simulink model "sampleModel1570_3"  (R2023a)
settings: Solver=VariableStepAuto  StartTime=0.0  StopTime=10.0  RelTol=1e-3
libraries: hdlsllib x8, simulink x3
settings Model: Creator=user1  LastModifiedBy=user1

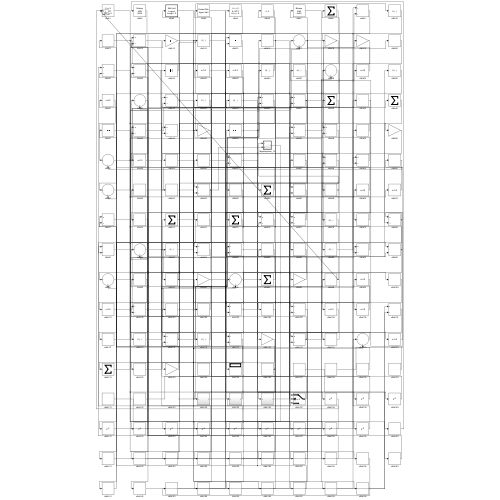
[thumbnail: Simulink's stored preview of the top-level diagram]
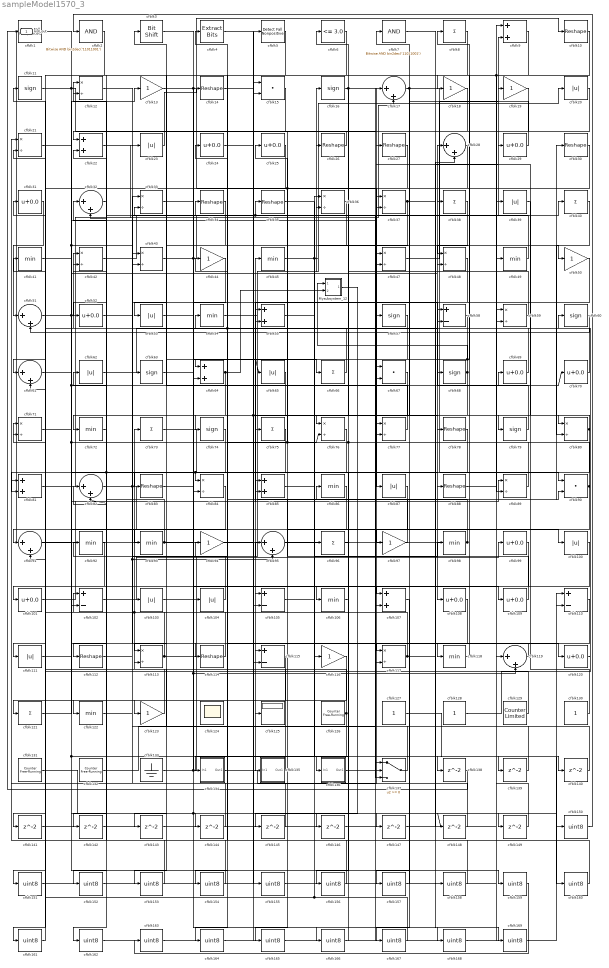
== system sampleModel1570_3 ==
  Mysubsystem_12 : Subsystem  TreatAsAtomicUnit=on  RTWFcnName=Mysubsystem_12
      settings: RTWFcnNameOpts=User specified  RTWFileNameOpts=Use function name
  cfblk1 : hdlsllib/Logic and Bit Operations/Detect Fall Nonpositive  vinit=0  OutDataTypeStr=uint8
  cfblk{10,14,26..27,30,34..35,78,83,88,112,114} (12 alike) : Reshape
  cfblk{20,23,39,53,62,65,87,100,103..104,111} (11 alike) : Abs  OutDataTypeStr=uint8  SaturateOnIntegerOverflow=off
  cfblk{24..25,29,31,52,69..70,99,101,108..109,120} (12 alike) : Bias  Bias=0.0  SaturateOnIntegerOverflow=off
  cfblk{58,102,105,110,115} (5 alike) : Sum  Inputs=+-  OutDataTypeStr=uint8
  cfblk{41,45,49,54,72,86,92..93,98,106,118,122} (12 alike) : MinMax  OutDataTypeStr=uint8
  cfblk{9,22,55,64,81,85,107} (7 alike) : Sum  OutDataTypeStr=uint8
  cfblk{11,16,57,60,63,68,74,79} (8 alike) : Signum
  cfblk{12,21,33,36..37,42..43,47..48,59,71,76..77,80,84,89,113,117} (18 alike) : Product  Inputs=*/  OutDataTypeStr=uint8  RndMeth=Zero  SaturateOnIntegerOverflow=on
  cfblk{13,18..19,44,50,94,97,116,123} (9 alike) : Gain  OutDataTypeStr=uint8
  cfblk{17,28,32,51,61,82,91,95,119} (9 alike) : Sum  Inputs=|++  OutDataTypeStr=uint8
  cfblk{8,38,40,66,73,75,96,121} (8 alike) : Sum  Inputs=+  OutDataTypeStr=uint8
  cfblk124 : Scope
      settings: Floating=on
  cfblk125 : Display
  cfblk126 : hdlsllib/Sources/Counter Free-Running  NumBits=16  tsamp=-1
  cfblk127 : Constant  OutDataTypeStr=uint8  SampleTime=-1
  cfblk128 : Constant  OutDataTypeStr=uint8  SampleTime=-1
  cfblk129 : hdlsllib/Sources/Counter Limited  uplimit=7  tsamp=-1
  cfblk130 : Constant  OutDataTypeStr=uint8  SampleTime=-1
  cfblk131 : hdlsllib/Sources/Counter Free-Running  NumBits=16  tsamp=-1
  cfblk132 : hdlsllib/Sources/Counter Free-Running  NumBits=16  tsamp=-1
  cfblk133 : Ground
  cfblk134 : Subsystem
      settings: LibrarySourceBlock=|
      | hdlsllib/Ports &
      | Subsystems/Subsystem
  cfblk135 : Subsystem
      settings: LibrarySourceBlock=|
      | hdlsllib/Ports &
      | Subsystems/Subsystem
  cfblk136 : Subsystem
      settings: LibrarySourceBlock=|
      | hdlsllib/Ports &
      | Subsystems/Subsystem
  cfblk137 : Switch  OutDataTypeStr=uint8  SaturateOnIntegerOverflow=off  InputSameDT=off
  cfblk{138..149} (12 alike) : Delay  SampleTime=1
  cfblk15 : DotProduct  OutDataTypeStr=uint8
  cfblk{150..169} (20 alike) : DataTypeConversion  OutDataTypeStr=uint8  SaturateOnIntegerOverflow=off  RndMeth=Floor
  cfblk2 : simulink/Logic and Bit Operations/Bitwise Operator  logicop=AND  UseBitMask=on  BitMask=bin2dec('11011001')  BitMaskRealWorld=Stored Integer
      settings: LibrarySourceBlock=|
      | hdlsllib/Logic and Bit
      | Operations/Bitwise
      | Operator
  cfblk3 : hdlsllib/Logic and Bit Operations/Bit Shift  mode=Shift Left Logical  N=0
  cfblk4 : simulink/Logic and Bit Operations/Extract Bits  bitsToExtract=Upper half  numBits=8  bitIdxRange=[0 7]  outScalingMode=Preserve fixed-point scaling
      settings: LibrarySourceBlock=|
      | hdlsllib/Logic and Bit
      | Operations/Extract Bits
  cfblk5 : hdlsllib/Logic and Bit Operations/Detect Fall Nonpositive  vinit=0  OutDataTypeStr=uint8
  cfblk6 : hdlsllib/Logic and Bit Operations/Compare To Constant  relop=<=  const=3.0  OutDataTypeStr=uint8
  cfblk67 : DotProduct  OutDataTypeStr=uint8
  cfblk7 : simulink/Logic and Bit Operations/Bitwise Operator  logicop=AND  UseBitMask=on  BitMask=bin2dec('11011001')  BitMaskRealWorld=Stored Integer
      settings: LibrarySourceBlock=|
      | hdlsllib/Logic and Bit
      | Operations/Bitwise
      | Operator
  cfblk90 : DotProduct  OutDataTypeStr=uint8
  Hdl_out : Outport  OutDataTypeStr=uint8
  wires:
  cfblk135/1(Out1) -> cfblk73/1
  cfblk134/1(Out1) -> cfblk17/1
  cfblk98/1 -> cfblk45/1, Hdl_out/1
  cfblk34/1 -> cfblk93/1
  cfblk29/1 -> cfblk64/1
  cfblk97/1 -> cfblk34/1
  cfblk75/1 -> cfblk82/2, cfblk91/1, cfblk84/1
  cfblk19/1 -> cfblk113/1
  cfblk17/1 -> cfblk90/1, cfblk77/1
  cfblk133/1 -> cfblk16/1, cfblk58/2
  cfblk101/1 -> cfblk89/1
  cfblk23/1 -> cfblk10/1
  cfblk13/1 -> cfblk87/1, cfblk137/2
  cfblk93/1 -> cfblk109/1, cfblk12/2
  cfblk45/1 -> cfblk50/1, cfblk78/1
  cfblk90/1 -> cfblk25/1, cfblk6/1, cfblk146/1
  cfblk48/1 -> cfblk135/1(In1)
  cfblk73/1 -> cfblk125/1
  cfblk128/1 -> cfblk80/1
  cfblk3/1 -> cfblk148/1, cfblk168/1, cfblk119/2
  cfblk49/1 -> cfblk35/1, cfblk12/1
  cfblk54/1 -> cfblk20/1
  cfblk99/1 -> cfblk101/1
  cfblk8/1 -> cfblk18/1
  cfblk43/1 -> cfblk9/2, cfblk37/1
  cfblk25/1 -> cfblk53/1
  cfblk89/1 -> cfblk4/1, cfblk55/2
  cfblk47/1 -> cfblk19/1
  cfblk83/1 -> cfblk14/1
  cfblk88/1 -> cfblk49/1
  cfblk113/1 -> cfblk103/1, cfblk91/2, cfblk26/1
  cfblk81/1 -> cfblk23/1
  cfblk39/1 -> cfblk79/1
  cfblk102/1 -> cfblk99/1
  cfblk79/1 -> cfblk28/1
  cfblk80/1 -> cfblk72/1, cfblk136/1(In1)
  cfblk26/1 -> cfblk22/1
  cfblk42/1 -> cfblk5/1
  cfblk110/1 -> cfblk167/1
  cfblk116/1 -> cfblk121/1
  cfblk52/1 -> cfblk118/1
  cfblk114/1 -> cfblk102/1
  cfblk20/1 -> cfblk89/2
  cfblk5/1 -> cfblk61/1
  cfblk115/1 -> cfblk122/1
  cfblk100/1 -> cfblk106/1
  cfblk95/1 -> cfblk69/1
  cfblk64/1 -> Mysubsystem_12/2(In2), cfblk112/1
  cfblk50/1 -> cfblk108/1
  cfblk78/1 -> cfblk111/1
  cfblk30/1 -> cfblk115/1, cfblk61/2
  cfblk31/1 -> cfblk51/1
  cfblk111/1 -> cfblk70/1, cfblk37/2
  cfblk10/1 -> cfblk68/1
  cfblk51/1 -> cfblk17/2, cfblk88/1, cfblk13/1
  cfblk33/1 -> cfblk66/1
  cfblk109/1 -> cfblk85/1
  cfblk82/1 -> cfblk115/2, cfblk120/1
  cfblk69/1 -> cfblk42/1
  cfblk62/1 -> cfblk57/1
  cfblk77/1 -> cfblk3/1
  cfblk24/1 -> cfblk107/1, cfblk77/2
  cfblk59/1 -> cfblk33/2
  cfblk37/1 -> cfblk84/2, cfblk29/1
  cfblk57/1 -> cfblk74/1
  cfblk119/1 -> cfblk117/1
  cfblk28/1 -> cfblk67/1
  cfblk35/1 -> cfblk116/1
  cfblk103/1 -> cfblk30/1
  cfblk44/1 -> cfblk64/2
  cfblk105/1 -> cfblk98/1
  cfblk132/1 -> cfblk47/1
  cfblk71/1 -> cfblk97/1, cfblk76/2
  cfblk76/1 -> cfblk81/2
  cfblk96/1 -> cfblk36/2
  cfblk65/1 -> cfblk83/1
  cfblk123/1 -> cfblk71/1
  cfblk68/1 -> Mysubsystem_12/1(In1), cfblk65/1, cfblk75/1
  cfblk12/1 -> cfblk63/1
  cfblk16/1 -> cfblk137/1, cfblk76/1
  cfblk60/1 -> cfblk51/2
  cfblk11/1 -> cfblk137/3, cfblk147/1, cfblk117/2
  cfblk40/1 -> cfblk80/2
  cfblk58/1 -> cfblk123/1
  cfblk129/1 -> cfblk71/2
  cfblk38/1 -> cfblk48/1
  cfblk18/1 -> cfblk55/1
  cfblk130/1 -> cfblk27/1
  cfblk104/1 -> cfblk92/1
  cfblk136/1(Out1) -> cfblk38/1
  cfblk70/1 -> cfblk41/1, cfblk44/1
  cfblk121/1 -> cfblk85/2
  cfblk63/1 -> cfblk104/1
  cfblk112/1 -> cfblk95/1
  cfblk117/1 -> cfblk42/2, cfblk90/2
  cfblk120/1 -> cfblk60/1
  cfblk1/1 -> cfblk43/2, cfblk114/1
  cfblk9/1 -> cfblk52/1, cfblk59/2
  cfblk126/1 -> cfblk134/1(In1), cfblk31/1
  cfblk87/1 -> cfblk105/1
  cfblk66/1 -> cfblk24/1
  cfblk61/1 -> cfblk48/2
  cfblk122/1 -> cfblk95/2, cfblk40/1
  cfblk118/1 -> cfblk8/1
  cfblk92/1 -> cfblk102/2
  cfblk137/1 -> cfblk54/1
  cfblk22/1 -> cfblk58/1
  cfblk91/1 -> cfblk100/1
  cfblk67/1 -> cfblk105/2
  cfblk55/1 -> cfblk138/1
  cfblk138/1 -> cfblk1/1
  cfblk85/1 -> cfblk139/1
  cfblk139/1 -> cfblk33/1
  cfblk4/1 -> cfblk140/1
  cfblk140/1 -> cfblk113/2
  cfblk84/1 -> cfblk141/1
  cfblk141/1 -> cfblk9/1
  cfblk72/1 -> cfblk142/1
  cfblk142/1 -> cfblk22/2
  cfblk36/1 -> cfblk143/1
  cfblk143/1 -> cfblk28/2
  cfblk41/1 -> cfblk144/1
  cfblk144/1 -> cfblk43/1
  cfblk145/1 -> cfblk81/1
  cfblk146/1 -> cfblk107/2
  cfblk148/1 -> cfblk82/1
  cfblk14/1 -> cfblk149/1
  cfblk149/1 -> cfblk59/1
  cfblk127/1 -> cfblk150/1
  cfblk150/1 -> cfblk2/1
  cfblk2/1 -> cfblk151/1
  cfblk151/1 -> cfblk119/1
  cfblk32/1 -> cfblk152/1
  cfblk152/1 -> cfblk96/1
  cfblk6/1 -> cfblk153/1
  cfblk153/1 -> cfblk32/1
  cfblk108/1 -> cfblk154/1
  cfblk154/1 -> cfblk32/2
  cfblk94/1 -> cfblk155/1
  cfblk155/1 -> cfblk67/2
  cfblk106/1 -> cfblk156/1
  cfblk156/1 -> cfblk94/1
  cfblk107/1 -> cfblk157/1
  cfblk157/1 -> cfblk7/1
  cfblk7/1 -> cfblk158/1
  cfblk158/1 -> cfblk62/1
  cfblk21/1 -> cfblk159/1
  cfblk131/1 -> cfblk160/1
  cfblk160/1 -> cfblk21/1
  cfblk74/1 -> cfblk161/1
  cfblk161/1 -> cfblk21/2
  cfblk15/1 -> cfblk162/1
  cfblk162/1 -> cfblk47/2
  cfblk159/1 -> cfblk163/1
  cfblk163/1 -> cfblk15/1
  cfblk27/1 -> cfblk164/1
  cfblk164/1 -> cfblk15/2
  cfblk86/1 -> cfblk165/1
  cfblk165/1 -> cfblk39/1
  cfblk53/1 -> cfblk166/1
  cfblk166/1 -> cfblk86/1
  cfblk167/1 -> cfblk11/1, cfblk36/1
  cfblk168/1 -> cfblk110/1
  cfblk147/1 -> cfblk169/1
  cfblk169/1 -> cfblk110/2
  Mysubsystem_12/1(Out1) -> cfblk145/1

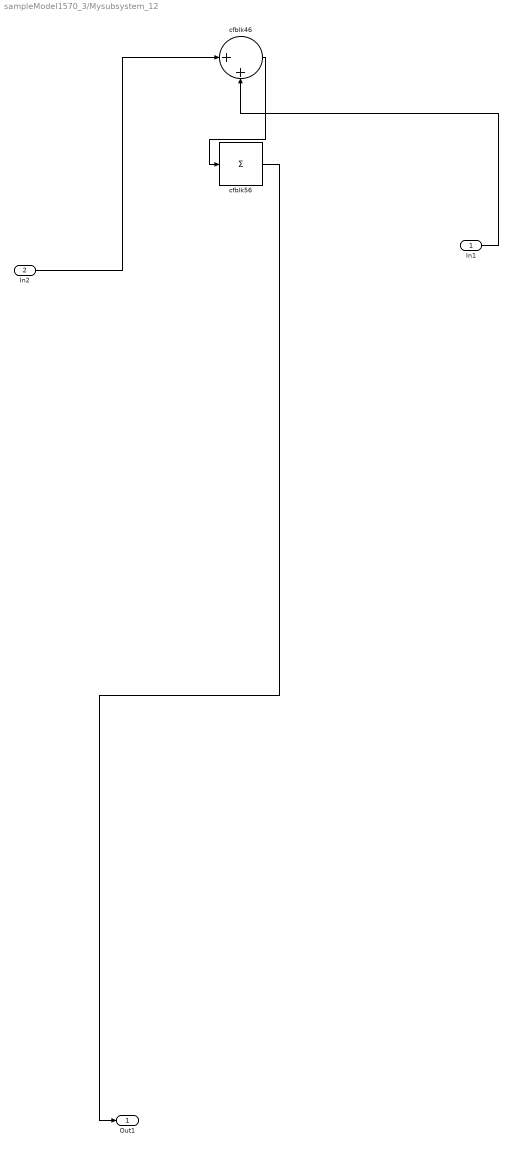
== system sampleModel1570_3/Mysubsystem_12 ==
  In1 : Inport
  In2 : Inport  Port=2
  cfblk46 : Sum  Inputs=|++
  cfblk56 : Sum  Inputs=+
  Out1 : Outport
  wires:
  cfblk46/1 -> cfblk56/1
  cfblk56/1 -> Out1/1
  In1/1 -> cfblk46/2
  In2/1 -> cfblk46/1

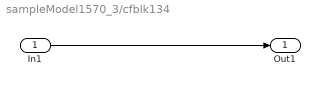
== system sampleModel1570_3/cfblk134 ==
  In1 : Inport
  Out1 : Outport
  wires:
  In1/1 -> Out1/1

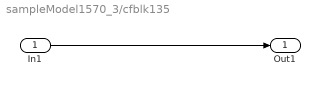
== system sampleModel1570_3/cfblk135 ==
  In1 : Inport
  Out1 : Outport
  wires:
  In1/1 -> Out1/1

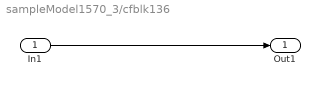
== system sampleModel1570_3/cfblk136 ==
  In1 : Inport
  Out1 : Outport
  wires:
  In1/1 -> Out1/1
